simulink model "e9_sf_slswitch"  (R2020a)
settings: Solver=FixedStepAuto  StartTime=0.0  StopTime=options.T_train  FixedStep=options.dt  MaxStep=.2  RelTol=1e-3
model workspace (MAT data in the model file):
  PID_TRESH = 0.3
undefined symbols (not defined in the file or in its folder): DiscIntNeverNeededParam, options
libraries: neural x72, simulink x3
(part 3 of 3)

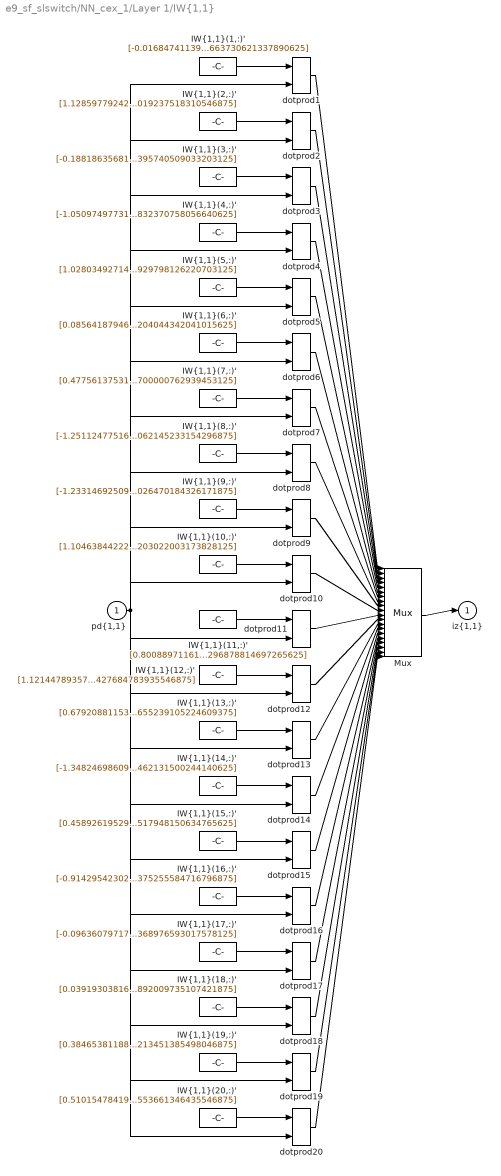
== system e9_sf_slswitch/NN_cex_1/Layer 1/IW{1,1} ==
  "pd{1,1}" : Inport  PortDimensions=6
      mask Display: e = 0.06;c1 = [120 230 180]/255;c2 = ([120 230 180]+0)/(256+128);c3 = ([120 230 180]+128)/(256+128);patch([0 1 1 0],[0 0 1 1],c1);patch([0 1 1 1-e 1-e 0+e],[0 0 1 1-e 0+e 0+e],c2);patch([0 0 1 1-e 0+e 0+e],[0 1 1 1-e 1-e 0+e],c3);plot([0 1 1 0 0],[0 0 1 1 0]);
  "IW{1,1}(1,:)'" : Constant  Value=[-0.0168474113906026019826800421697043930180370807647705078125;-1.0960190446116688800515248658484779298305511474609375;1.303822159020755488967324708937667310237884521484375;0.90483138367543614055676926000160165131092071533203125;-0.92904857435732768333735975829767994582653045654296875;0.7536625946512780505059936331235803663730621337890625]
      mask Display: e = 0.06;c1 = [120 150 230]/255;c2 = ([120 150 230]+0)/383;c3 = ([120 150 230]+128)/383;patch([0 1 1 0],[0 0 1 1],c1);patch([0 1 1 1-e 1-e 0+e],[0 0 1 1-e 0+e 0+e],c2);patch([0 0 1 1-e 0+e 0+e],[0 1 1 1-e 1-e 0+e],c3);plot([0 1 1 0 0],[0 0 1 1 0]);disp('Weights');
  "IW{1,1}(10,:)'" : Constant  Value=[1.104638442227569239406648193835280835628509521484375;-0.02443218271199705526885992412644554860889911651611328125;-0.54301394151020698775056416707229800522327423095703125;-2.64487319649380747677014369401149451732635498046875;0.83816378231433186218879427542560733854770660400390625;0.580117155258321748334537915070541203022003173828125]
      mask Display: e = 0.06;c1 = [120 150 230]/255;c2 = ([120 150 230]+0)/383;c3 = ([120 150 230]+128)/383;patch([0 1 1 0],[0 0 1 1],c1);patch([0 1 1 1-e 1-e 0+e],[0 0 1 1-e 0+e 0+e],c2);patch([0 0 1 1-e 0+e 0+e],[0 1 1 1-e 1-e 0+e],c3);plot([0 1 1 0 0],[0 0 1 1 0]);disp('Weights');
  "IW{1,1}(11,:)'" : Constant  Value=[0.80088971161301392154285849755979143083095550537109375;-1.4360458039470860303055133044836111366748809814453125;1.349244522904669896234963744063861668109893798828125;0.239507763293771269719201200132374651730060577392578125;-0.142625375011002863967490839058882556855678558349609375;-1.1145437179066368660329544582054950296878814697265625]
      mask Display: e = 0.06;c1 = [120 150 230]/255;c2 = ([120 150 230]+0)/383;c3 = ([120 150 230]+128)/383;patch([0 1 1 0],[0 0 1 1],c1);patch([0 1 1 1-e 1-e 0+e],[0 0 1 1-e 0+e 0+e],c2);patch([0 0 1 1-e 0+e 0+e],[0 1 1 1-e 1-e 0+e],c3);plot([0 1 1 0 0],[0 0 1 1 0]);disp('Weights');
  "IW{1,1}(12,:)'" : Constant  Value=[1.12144789357198959578454378060996532440185546875;-1.039431996259746693311853960040025413036346435546875;-0.06963854228211265040560107308920123614370822906494140625;-0.388663791726383378577480698368162848055362701416015625;-0.526178830323278834413258664426393806934356689453125;1.8227062352942435818903277322533540427684783935546875]
      mask Display: e = 0.06;c1 = [120 150 230]/255;c2 = ([120 150 230]+0)/383;c3 = ([120 150 230]+128)/383;patch([0 1 1 0],[0 0 1 1],c1);patch([0 1 1 1-e 1-e 0+e],[0 0 1 1-e 0+e 0+e],c2);patch([0 0 1 1-e 0+e 0+e],[0 1 1 1-e 1-e 0+e],c3);plot([0 1 1 0 0],[0 0 1 1 0]);disp('Weights');
  "IW{1,1}(13,:)'" : Constant  Value=[0.6792088115375027879139224751270376145839691162109375;-0.67422879238008082136701659692334942519664764404296875;1.1697043443831096620755261028534732758998870849609375;-0.5713364836554226666720524008269421756267547607421875;-1.3593652703803027481654908115160651504993438720703125;-0.67325667405921796326850881087011657655239105224609375]
      mask Display: e = 0.06;c1 = [120 150 230]/255;c2 = ([120 150 230]+0)/383;c3 = ([120 150 230]+128)/383;patch([0 1 1 0],[0 0 1 1],c1);patch([0 1 1 1-e 1-e 0+e],[0 0 1 1-e 0+e 0+e],c2);patch([0 0 1 1-e 0+e 0+e],[0 1 1 1-e 1-e 0+e],c3);plot([0 1 1 0 0],[0 0 1 1 0]);disp('Weights');
  "IW{1,1}(14,:)'" : Constant  Value=[-1.348246986096783839315094155608676373958587646484375;0.007208702054189595510858001858878196799196302890777587890625;0.689323370229841803080716999829746782779693603515625;0.274921664510416829951822137445560656487941741943359375;0.9517793019769207329972005027229897677898406982421875;1.4034991564643990447081023376085795462131500244140625]
      mask Display: e = 0.06;c1 = [120 150 230]/255;c2 = ([120 150 230]+0)/383;c3 = ([120 150 230]+128)/383;patch([0 1 1 0],[0 0 1 1],c1);patch([0 1 1 1-e 1-e 0+e],[0 0 1 1-e 0+e 0+e],c2);patch([0 0 1 1-e 0+e 0+e],[0 1 1 1-e 1-e 0+e],c3);plot([0 1 1 0 0],[0 0 1 1 0]);disp('Weights');
  "IW{1,1}(15,:)'" : Constant  Value=[0.458926195297770345149501736159436404705047607421875;-0.82721661614949237861793562842649407684803009033203125;-1.0472964443914991594652974526979960501194000244140625;2.286396458456293689920357792288996279239654541015625;-0.767283880026006226415802302653901278972625732421875;-1.2787583371301727286351024304167367517948150634765625]
      mask Display: e = 0.06;c1 = [120 150 230]/255;c2 = ([120 150 230]+0)/383;c3 = ([120 150 230]+128)/383;patch([0 1 1 0],[0 0 1 1],c1);patch([0 1 1 1-e 1-e 0+e],[0 0 1 1-e 0+e 0+e],c2);patch([0 0 1 1-e 0+e 0+e],[0 1 1 1-e 1-e 0+e],c3);plot([0 1 1 0 0],[0 0 1 1 0]);disp('Weights');
  "IW{1,1}(16,:)'" : Constant  Value=[-0.9142954230218294231491427126456983387470245361328125;1.086582668659030304070256534032523632049560546875;-0.5623194252036516349591011021402664482593536376953125;0.9130879165472227665389937101281248033046722412109375;-0.378624198635671704860072850351571105420589447021484375;1.1245605733918313529073884637909941375255584716796875]
      mask Display: e = 0.06;c1 = [120 150 230]/255;c2 = ([120 150 230]+0)/383;c3 = ([120 150 230]+128)/383;patch([0 1 1 0],[0 0 1 1],c1);patch([0 1 1 1-e 1-e 0+e],[0 0 1 1-e 0+e 0+e],c2);patch([0 0 1 1-e 0+e 0+e],[0 1 1 1-e 1-e 0+e],c3);plot([0 1 1 0 0],[0 0 1 1 0]);disp('Weights');
  "IW{1,1}(17,:)'" : Constant  Value=[-0.0963607971765284287979369537424645386636257171630859375;0.52383887892794100960003333966596983373165130615234375;1.1199200021715942643396601852145977318286895751953125;0.412214510505207132329275054871686734259128570556640625;1.493814360897363968661011313088238239288330078125;1.0969306752620930911490404469077475368976593017578125]
      mask Display: e = 0.06;c1 = [120 150 230]/255;c2 = ([120 150 230]+0)/383;c3 = ([120 150 230]+128)/383;patch([0 1 1 0],[0 0 1 1],c1);patch([0 1 1 1-e 1-e 0+e],[0 0 1 1-e 0+e 0+e],c2);patch([0 0 1 1-e 0+e 0+e],[0 1 1 1-e 1-e 0+e],c3);plot([0 1 1 0 0],[0 0 1 1 0]);disp('Weights');
  "IW{1,1}(18,:)'" : Constant  Value=[0.03919303816683929186925894327941932715475559234619140625;-1.705405108377961109766829395084641873836517333984375;1.4225063236010502265571631141938269138336181640625;0.74230993989574856062318986005266197025775909423828125;0.03172256129110760658473822104497230611741542816162109375;-0.64635944684935520143653775448910892009735107421875]
      mask Display: e = 0.06;c1 = [120 150 230]/255;c2 = ([120 150 230]+0)/383;c3 = ([120 150 230]+128)/383;patch([0 1 1 0],[0 0 1 1],c1);patch([0 1 1 1-e 1-e 0+e],[0 0 1 1-e 0+e 0+e],c2);patch([0 0 1 1-e 0+e 0+e],[0 1 1 1-e 1-e 0+e],c3);plot([0 1 1 0 0],[0 0 1 1 0]);disp('Weights');
  "IW{1,1}(19,:)'" : Constant  Value=[0.38465381188996261574430945984204299747943878173828125;-1.3456866197282078001506988584878854453563690185546875;1.0543182684732188558740517692058347165584564208984375;-1.09418022738094578016898594796657562255859375;0.381893554029432202856497724496875889599323272705078125;-0.96869250594760980543895811933907680213451385498046875]
      mask Display: e = 0.06;c1 = [120 150 230]/255;c2 = ([120 150 230]+0)/383;c3 = ([120 150 230]+128)/383;patch([0 1 1 0],[0 0 1 1],c1);patch([0 1 1 1-e 1-e 0+e],[0 0 1 1-e 0+e 0+e],c2);patch([0 0 1 1-e 0+e 0+e],[0 1 1 1-e 1-e 0+e],c3);plot([0 1 1 0 0],[0 0 1 1 0]);disp('Weights');
  "IW{1,1}(2,:)'" : Constant  Value=[1.1285977924294738894417378105572424829006195068359375;1.3719496232898198417871071796980686485767364501953125;-0.70013930920313305339419684969470836222171783447265625;-0.40779886428615153004528792735072784125804901123046875;-1.3652168438495941860111315691028721630573272705078125;-2.669548479833547371953272886457853019237518310546875]
      mask Display: e = 0.06;c1 = [120 150 230]/255;c2 = ([120 150 230]+0)/383;c3 = ([120 150 230]+128)/383;patch([0 1 1 0],[0 0 1 1],c1);patch([0 1 1 1-e 1-e 0+e],[0 0 1 1-e 0+e 0+e],c2);patch([0 0 1 1-e 0+e 0+e],[0 1 1 1-e 1-e 0+e],c3);plot([0 1 1 0 0],[0 0 1 1 0]);disp('Weights');
  "IW{1,1}(20,:)'" : Constant  Value=[0.51015478419691684397463404820882715284824371337890625;-0.797711507045957279871117862057872116565704345703125;-0.51591444607071179628832169328234158456325531005859375;-1.3440860874112698919446984291425906121730804443359375;1.16622740943395086787859327159821987152099609375;-1.0335932152524047733521683767321519553661346435546875]
      mask Display: e = 0.06;c1 = [120 150 230]/255;c2 = ([120 150 230]+0)/383;c3 = ([120 150 230]+128)/383;patch([0 1 1 0],[0 0 1 1],c1);patch([0 1 1 1-e 1-e 0+e],[0 0 1 1-e 0+e 0+e],c2);patch([0 0 1 1-e 0+e 0+e],[0 1 1 1-e 1-e 0+e],c3);plot([0 1 1 0 0],[0 0 1 1 0]);disp('Weights');
  "IW{1,1}(3,:)'" : Constant  Value=[-0.188186356814592503639005371951498091220855712890625;0.04608541339057010965962746240620617754757404327392578125;0.477858638180441774867546200766810216009616851806640625;-1.008508128728536679119542895932681858539581298828125;-1.2120727840960991983365602209232747554779052734375;-1.125534165151560461737290097516961395740509033203125]
      mask Display: e = 0.06;c1 = [120 150 230]/255;c2 = ([120 150 230]+0)/383;c3 = ([120 150 230]+128)/383;patch([0 1 1 0],[0 0 1 1],c1);patch([0 1 1 1-e 1-e 0+e],[0 0 1 1-e 0+e 0+e],c2);patch([0 0 1 1-e 0+e 0+e],[0 1 1 1-e 1-e 0+e],c3);plot([0 1 1 0 0],[0 0 1 1 0]);disp('Weights');
  "IW{1,1}(4,:)'" : Constant  Value=[-1.050974977312110869576144978054799139499664306640625;1.28629718055694386436016429797746241092681884765625;1.1326800600668465168752163663157261908054351806640625;-0.82019920554920144883936927726608701050281524658203125;0.13774083756492638830337682520621456205844879150390625;-0.7371803862906036730606729179271496832370758056640625]
      mask Display: e = 0.06;c1 = [120 150 230]/255;c2 = ([120 150 230]+0)/383;c3 = ([120 150 230]+128)/383;patch([0 1 1 0],[0 0 1 1],c1);patch([0 1 1 1-e 1-e 0+e],[0 0 1 1-e 0+e 0+e],c2);patch([0 0 1 1-e 0+e 0+e],[0 1 1 1-e 1-e 0+e],c3);plot([0 1 1 0 0],[0 0 1 1 0]);disp('Weights');
  "IW{1,1}(5,:)'" : Constant  Value=[1.0280349271452358106415658767218701541423797607421875;0.402195825930382111490501984008005820214748382568359375;-1.241108396864921470381659673876129090785980224609375;-1.0859758989406571583202776309917680919170379638671875;-0.98306862033537123490845033302321098744869232177734375;0.1483100282919010137749893374348175711929798126220703125]
      mask Display: e = 0.06;c1 = [120 150 230]/255;c2 = ([120 150 230]+0)/383;c3 = ([120 150 230]+128)/383;patch([0 1 1 0],[0 0 1 1],c1);patch([0 1 1 1-e 1-e 0+e],[0 0 1 1-e 0+e 0+e],c2);patch([0 0 1 1-e 0+e 0+e],[0 1 1 1-e 1-e 0+e],c3);plot([0 1 1 0 0],[0 0 1 1 0]);disp('Weights');
  "IW{1,1}(6,:)'" : Constant  Value=[0.08564187946235080062251654453575611114501953125;-1.0587143232822635585677062408649362623691558837890625;0.99533659624054260373071656431420706212520599365234375;1.348286797369088407805293172714300453662872314453125;-0.75350782154291906511645038335700519382953643798828125;-1.4647900005101688325481745778233744204044342041015625]
      mask Display: e = 0.06;c1 = [120 150 230]/255;c2 = ([120 150 230]+0)/383;c3 = ([120 150 230]+128)/383;patch([0 1 1 0],[0 0 1 1],c1);patch([0 1 1 1-e 1-e 0+e],[0 0 1 1-e 0+e 0+e],c2);patch([0 0 1 1-e 0+e 0+e],[0 1 1 1-e 1-e 0+e],c3);plot([0 1 1 0 0],[0 0 1 1 0]);disp('Weights');
  "IW{1,1}(7,:)'" : Constant  Value=[0.477561375317118452787923388314084149897098541259765625;-1.422656231024767681248022199724800884723663330078125;-0.34547470258236157025777401941013522446155548095703125;-0.6180573185750326548060229470138438045978546142578125;-1.103280002866290576690744273946620523929595947265625;-0.77979501040747056794799618728575296700000762939453125]
      mask Display: e = 0.06;c1 = [120 150 230]/255;c2 = ([120 150 230]+0)/383;c3 = ([120 150 230]+128)/383;patch([0 1 1 0],[0 0 1 1],c1);patch([0 1 1 1-e 1-e 0+e],[0 0 1 1-e 0+e 0+e],c2);patch([0 0 1 1-e 0+e 0+e],[0 1 1 1-e 1-e 0+e],c3);plot([0 1 1 0 0],[0 0 1 1 0]);disp('Weights');
  "IW{1,1}(8,:)'" : Constant  Value=[-1.251124775166029490236496712896041572093963623046875;1.0049111421650123165960621918202377855777740478515625;0.77937459336890635430705742692225612699985504150390625;-0.82407450496222856006767187864170409739017486572265625;0.380603729542155100329381411938811652362346649169921875;-1.18248664285082139002724943566136062145233154296875]
      mask Display: e = 0.06;c1 = [120 150 230]/255;c2 = ([120 150 230]+0)/383;c3 = ([120 150 230]+128)/383;patch([0 1 1 0],[0 0 1 1],c1);patch([0 1 1 1-e 1-e 0+e],[0 0 1 1-e 0+e 0+e],c2);patch([0 0 1 1-e 0+e 0+e],[0 1 1 1-e 1-e 0+e],c3);plot([0 1 1 0 0],[0 0 1 1 0]);disp('Weights');
  "IW{1,1}(9,:)'" : Constant  Value=[-1.2331469250970192863547936212853528559207916259765625;-0.2645454198128656120303503485047258436679840087890625;0.28872687215204162480830518688890151679515838623046875;-0.91218425882033937757142894042772240936756134033203125;-0.382274517593333584830617155603249557316303253173828125;1.50022977818130254235029497067444026470184326171875]
      mask Display: e = 0.06;c1 = [120 150 230]/255;c2 = ([120 150 230]+0)/383;c3 = ([120 150 230]+128)/383;patch([0 1 1 0],[0 0 1 1],c1);patch([0 1 1 1-e 1-e 0+e],[0 0 1 1-e 0+e 0+e],c2);patch([0 0 1 1-e 0+e 0+e],[0 1 1 1-e 1-e 0+e],c3);plot([0 1 1 0 0],[0 0 1 1 0]);disp('Weights');
  Mux : Mux  Inputs=20
      mask Display: e = 0.06;c1 = [120 150 230]/255;c2 = ([120 150 230]+0)/383;c3 = ([120 150 230]+128)/383;patch([0 1 1 0],[0 0 1 1],c1);patch([0 1 1 1-e 1-e 0+e],[0 0 1 1-e 0+e 0+e],c2);patch([0 0 1 1-e 0+e 0+e],[0 1 1 1-e 1-e 0+e],c3);plot([0 1 1 0 0],[0 0 1 1 0]);disp('Mux');
  dotprod{1..20} (20 alike) : neural/Weight Functions/dotprod
  "iz{1,1}" : Outport
      mask Display: e = 0.06;c1 = [120 230 180]/255;c2 = ([120 230 180]+0)/(256+128);c3 = ([120 230 180]+128)/(256+128);patch([0 1 1 0],[0 0 1 1],c1);patch([0 1 1 1-e 1-e 0+e],[0 0 1 1-e 0+e 0+e],c2);patch([0 0 1 1-e 0+e 0+e],[0 1 1 1-e 1-e 0+e],c3);plot([0 1 1 0 0],[0 0 1 1 0]);
  wires:
  "IW{1,1}(1,:)'"/1 -> dotprod1/1
  "pd{1,1}"/1 -> dotprod1/2, dotprod2/2, dotprod3/2, dotprod4/2, dotprod5/2, dotprod6/2, dotprod7/2, dotprod8/2, dotprod9/2, dotprod10/2, dotprod11/2, dotprod12/2, dotprod13/2, dotprod14/2, dotprod15/2, dotprod16/2, dotprod17/2, dotprod18/2, dotprod19/2, dotprod20/2
  dotprod1/1 -> Mux/1
  "IW{1,1}(2,:)'"/1 -> dotprod2/1
  dotprod2/1 -> Mux/2
  "IW{1,1}(3,:)'"/1 -> dotprod3/1
  dotprod3/1 -> Mux/3
  "IW{1,1}(4,:)'"/1 -> dotprod4/1
  dotprod4/1 -> Mux/4
  "IW{1,1}(5,:)'"/1 -> dotprod5/1
  dotprod5/1 -> Mux/5
  "IW{1,1}(6,:)'"/1 -> dotprod6/1
  dotprod6/1 -> Mux/6
  "IW{1,1}(7,:)'"/1 -> dotprod7/1
  dotprod7/1 -> Mux/7
  "IW{1,1}(8,:)'"/1 -> dotprod8/1
  dotprod8/1 -> Mux/8
  "IW{1,1}(9,:)'"/1 -> dotprod9/1
  dotprod9/1 -> Mux/9
  "IW{1,1}(10,:)'"/1 -> dotprod10/1
  dotprod10/1 -> Mux/10
  "IW{1,1}(11,:)'"/1 -> dotprod11/1
  dotprod11/1 -> Mux/11
  "IW{1,1}(12,:)'"/1 -> dotprod12/1
  dotprod12/1 -> Mux/12
  "IW{1,1}(13,:)'"/1 -> dotprod13/1
  dotprod13/1 -> Mux/13
  "IW{1,1}(14,:)'"/1 -> dotprod14/1
  dotprod14/1 -> Mux/14
  "IW{1,1}(15,:)'"/1 -> dotprod15/1
  dotprod15/1 -> Mux/15
  "IW{1,1}(16,:)'"/1 -> dotprod16/1
  dotprod16/1 -> Mux/16
  "IW{1,1}(17,:)'"/1 -> dotprod17/1
  dotprod17/1 -> Mux/17
  "IW{1,1}(18,:)'"/1 -> dotprod18/1
  dotprod18/1 -> Mux/18
  "IW{1,1}(19,:)'"/1 -> dotprod19/1
  dotprod19/1 -> Mux/19
  "IW{1,1}(20,:)'"/1 -> dotprod20/1
  dotprod20/1 -> Mux/20
  Mux/1 -> "iz{1,1}"/1

== system e9_sf_slswitch/NN_cex_1/Layer 2/Delays 1 ==
  "p{2}" : Inport  PortDimensions=20
      mask Display: e = 0.06;c1 = [120 230 180]/255;c2 = ([120 230 180]+0)/(256+128);c3 = ([120 230 180]+128)/(256+128);patch([0 1 1 0],[0 0 1 1],c1);patch([0 1 1 1-e 1-e 0+e],[0 0 1 1-e 0+e 0+e],c2);patch([0 0 1 1-e 0+e 0+e],[0 1 1 1-e 1-e 0+e],c3);plot([0 1 1 0 0],[0 0 1 1 0]);
  mux : Mux  Inputs=1
      mask Display: e = 0.06;c1 = [120 150 230]/255;c2 = ([120 150 230]+0)/383;c3 = ([120 150 230]+128)/383;patch([0 1 1 0],[0 0 1 1],c1);patch([0 1 1 1-e 1-e 0+e],[0 0 1 1-e 0+e 0+e],c2);patch([0 0 1 1-e 0+e 0+e],[0 1 1 1-e 1-e 0+e],c3);plot([0 1 1 0 0],[0 0 1 1 0]);disp('Mux')
  "pd{2,1}" : Outport
      mask Display: e = 0.06;c1 = [120 230 180]/255;c2 = ([120 230 180]+0)/(256+128);c3 = ([120 230 180]+128)/(256+128);patch([0 1 1 0],[0 0 1 1],c1);patch([0 1 1 1-e 1-e 0+e],[0 0 1 1-e 0+e 0+e],c2);patch([0 0 1 1-e 0+e 0+e],[0 1 1 1-e 1-e 0+e],c3);plot([0 1 1 0 0],[0 0 1 1 0]);
  wires:
  "p{2}"/1 -> mux/1
  mux/1 -> "pd{2,1}"/1

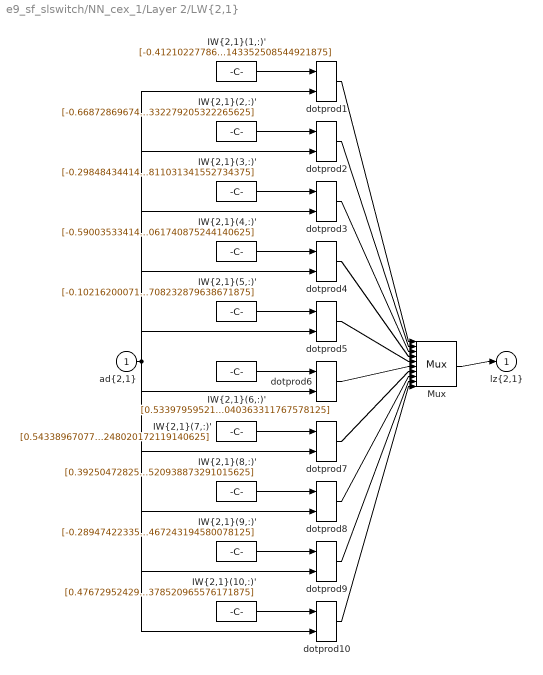
== system e9_sf_slswitch/NN_cex_1/Layer 2/LW{2,1} ==
  "ad{2,1}" : Inport  PortDimensions=20
      mask Display: e = 0.06;c1 = [120 230 180]/255;c2 = ([120 230 180]+0)/(256+128);c3 = ([120 230 180]+128)/(256+128);patch([0 1 1 0],[0 0 1 1],c1);patch([0 1 1 1-e 1-e 0+e],[0 0 1 1-e 0+e 0+e],c2);patch([0 0 1 1-e 0+e 0+e],[0 1 1 1-e 1-e 0+e],c3);plot([0 1 1 0 0],[0 0 1 1 0]);
  "IW{2,1}(1,:)'" : Constant  Value=[-0.412102277869951072464260732886032201349735260009765625;-0.0033102962537368790622849257232473973999731242656707763671875;0.498276475510173455507612061410327441990375518798828125;0.370594648987040031773432247064192779362201690673828125;-0.172702581187572423715437253122217953205108642578125;-0.28269873284898405785270369960926473140716552734375;0.1609017986261900567956928398416494019329547882080078125;0.57527437877796694376542063764645718038082122802734375;0.18571656848820394802856981186778284609317779541015625;-0.397447810976002013916286159656010568141937255859375;-0.49313231453008621318900850383215583860874176025390625;-0.3183651289608493417659929036744870245456695556640625;0.1503184907699568750860663612911594100296497344970703125;-0.343042617011638795165850979174138046801090240478515625;0.48159614366312475386422420342569239437580108642578125;-0.384340370033912359648553547231131233274936676025390625;0.319803972642864697828457565265125595033168792724609375;-0.169210525256166477436892137120594270527362823486328125;0.1082045460649214974058196503392537124454975128173828125;0.49225160804730883068458524576271884143352508544921875]
      mask Display: e = 0.06;c1 = [120 150 230]/255;c2 = ([120 150 230]+0)/383;c3 = ([120 150 230]+128)/383;patch([0 1 1 0],[0 0 1 1],c1);patch([0 1 1 1-e 1-e 0+e],[0 0 1 1-e 0+e 0+e],c2);patch([0 0 1 1-e 0+e 0+e],[0 1 1 1-e 1-e 0+e],c3);plot([0 1 1 0 0],[0 0 1 1 0]);disp('weights');
  "IW{2,1}(10,:)'" : Constant  Value=[0.476729524297248519193459515008726157248020172119140625;-0.407821347083386298582041717963875271379947662353515625;-0.2018949387792945693309576427054707892239093780517578125;-0.4059574043654183839180404902435839176177978515625;0.73472791573249873753326255609863437712192535400390625;0.511372507461387737492941596428863704204559326171875;0.69961983003993666319075828141649253666400909423828125;-0.234222692241623675624140332729439251124858856201171875;0.19033737019719054739397279263357631862163543701171875;-0.2296240379397176400999569523264653980731964111328125;0.52125524089998609422735853513586334884166717529296875;-0.95321599331459638815289281410514377057552337646484375;0.1506847813854093887098173354388563893735408782958984375;0.51547730872195796081314256298355758190155029296875;0.274123361606459725603457400211482308804988861083984375;0.1863257308692378988457249988641706295311450958251953125;-0.5345344958086812869879622667212970554828643798828125;0.2183490567687410288666427504722378216683864593505859375;-0.215592460422616927218086857465095818042755126953125;0.0175481619752120114597015998469942132942378520965576171875]
      mask Display: e = 0.06;c1 = [120 150 230]/255;c2 = ([120 150 230]+0)/383;c3 = ([120 150 230]+128)/383;patch([0 1 1 0],[0 0 1 1],c1);patch([0 1 1 1-e 1-e 0+e],[0 0 1 1-e 0+e 0+e],c2);patch([0 0 1 1-e 0+e 0+e],[0 1 1 1-e 1-e 0+e],c3);plot([0 1 1 0 0],[0 0 1 1 0]);disp('weights');
  "IW{2,1}(2,:)'" : Constant  Value=[-0.6687286967479215693543892484740354120731353759765625;0.53089310457156846378978798384196124970912933349609375;-0.00988650741851515406366512905833587865345180034637451171875;-0.16475866593556764971850725487456656992435455322265625;-0.83099792149795803641865177269210107624530792236328125;0.83286438268544260576931037576287053525447845458984375;-0.421930961865297604607150105948676355183124542236328125;0.06684041765297595028005872563880984671413898468017578125;-0.173504636537880951863144218805246055126190185546875;0.1793284238400363606036336250326712615787982940673828125;-0.412807134717095181031254469417035579681396484375;-0.1897621024386075549994501443507033400237560272216796875;0.1393131970130082886161204669406288303434848785400390625;0.1878438569324507312341410170120070688426494598388671875;0.86404371044378092125981538629275746643543243408203125;0.46470926606683515824869346033665351569652557373046875;0.038250058996138480704729545323061756789684295654296875;0.221752079748374464340798795092268846929073333740234375;0.192947140226262359163911241921596229076385498046875;-0.349200177440924852678705292419181205332279205322265625]
      mask Display: e = 0.06;c1 = [120 150 230]/255;c2 = ([120 150 230]+0)/383;c3 = ([120 150 230]+128)/383;patch([0 1 1 0],[0 0 1 1],c1);patch([0 1 1 1-e 1-e 0+e],[0 0 1 1-e 0+e 0+e],c2);patch([0 0 1 1-e 0+e 0+e],[0 1 1 1-e 1-e 0+e],c3);plot([0 1 1 0 0],[0 0 1 1 0]);disp('weights');
  "IW{2,1}(3,:)'" : Constant  Value=[-0.298484344147023239468552446851390413939952850341796875;0.190641928235647295508670140407048165798187255859375;0.1981536900428658432016248980289674364030361175537109375;-0.388862957242743612074065140404854901134967803955078125;0.21449537302792165416320813164929859340190887451171875;0.3863203233730050367711328362929634749889373779296875;0.68170524276259214513373763111303560435771942138671875;0.12950440289639064683768765462446026504039764404296875;0.327443722942501846961960154658299870789051055908203125;-0.542516816538905377598211998702026903629302978515625;0.3702632632852640437448599186609499156475067138671875;-0.262759426109619109723780638887546956539154052734375;0.398897950183966065740293061026022769510746002197265625;-0.2405628118556803751726391737975063733756542205810546875;-0.418319523738042098326417317366576753556728363037109375;-0.057500676569799409609817786304120090790092945098876953125;0.432838580152064944517320554950856603682041168212890625;0.406924514266054526689941894801449961960315704345703125;0.2437061579769842223353037979904911480844020843505859375;-0.451417764465296522669035539365722797811031341552734375]
      mask Display: e = 0.06;c1 = [120 150 230]/255;c2 = ([120 150 230]+0)/383;c3 = ([120 150 230]+128)/383;patch([0 1 1 0],[0 0 1 1],c1);patch([0 1 1 1-e 1-e 0+e],[0 0 1 1-e 0+e 0+e],c2);patch([0 0 1 1-e 0+e 0+e],[0 1 1 1-e 1-e 0+e],c3);plot([0 1 1 0 0],[0 0 1 1 0]);disp('weights');
  "IW{2,1}(4,:)'" : Constant  Value=[-0.590035334144344947304716697544790804386138916015625;-0.14251153895537560511996844070381484925746917724609375;0.055844163610838937206182208683458156883716583251953125;-0.25168425456298348930062047656974755227565765380859375;0.347940176225571440316031157635734416544437408447265625;0.334331889113240132704873985858284868299961090087890625;-0.3570468479858923682712656955118291079998016357421875;-0.487904252695575468834476851043291389942169189453125;0.066019736601342859927399331354536116123199462890625;0.09407698569578033798155303202292998321354389190673828125;-0.2450555949832949609312748862066655419766902923583984375;0.36422969241255109817956281403894536197185516357421875;-0.3245571948522207872400713313254527747631072998046875;0.64482395367362543847633560289978049695491790771484375;0.137767167812864410603168607849511317908763885498046875;0.429727741927319495385262371200951747596263885498046875;-0.043270745376913381796679658464199746958911418914794921875;0.14654430233835558095023543501156382262706756591796875;0.47476898943911083339486367549397982656955718994140625;0.55073672846336096942110316376783885061740875244140625]
      mask Display: e = 0.06;c1 = [120 150 230]/255;c2 = ([120 150 230]+0)/383;c3 = ([120 150 230]+128)/383;patch([0 1 1 0],[0 0 1 1],c1);patch([0 1 1 1-e 1-e 0+e],[0 0 1 1-e 0+e 0+e],c2);patch([0 0 1 1-e 0+e 0+e],[0 1 1 1-e 1-e 0+e],c3);plot([0 1 1 0 0],[0 0 1 1 0]);disp('weights');
  "IW{2,1}(5,:)'" : Constant  Value=[-0.1021620007108376970705876374267973005771636962890625;0.43940207024349131614826546865515410900115966796875;0.420315012299466383982604611446731723845005035400390625;-0.268809769837709711115536492798128165304660797119140625;-0.66491121568533506636100582909421063959598541259765625;0.81368602130842127007070985200698487460613250732421875;-0.0209290057054771945488358397824413259513676166534423828125;0.60030318645803582011666321704979054629802703857421875;0.05965638396169337109853358924738131463527679443359375;0.46479724467141825261506937749800272285938262939453125;-0.49210398709284419727083559337188489735126495361328125;-0.256405350236701135013817065555485896766185760498046875;0.2117572317136166837325816914017195813357830047607421875;0.0665783902974867725088614633932593278586864471435546875;-0.5574717002200204607476052842685021460056304931640625;-0.2042746665310815334937188936237362213432788848876953125;-0.3718070675272440173131371921044774353504180908203125;0.1607832109368834971885320328510715626180171966552734375;-0.09600919695738129033824037605882040224969387054443359375;-0.05362222814658224034900513288448564708232879638671875]
      mask Display: e = 0.06;c1 = [120 150 230]/255;c2 = ([120 150 230]+0)/383;c3 = ([120 150 230]+128)/383;patch([0 1 1 0],[0 0 1 1],c1);patch([0 1 1 1-e 1-e 0+e],[0 0 1 1-e 0+e 0+e],c2);patch([0 0 1 1-e 0+e 0+e],[0 1 1 1-e 1-e 0+e],c3);plot([0 1 1 0 0],[0 0 1 1 0]);disp('weights');
  "IW{2,1}(6,:)'" : Constant  Value=[0.533979595219758795821007879567332565784454345703125;0.4951544592086138951714247014024294912815093994140625;0.386181435740664991129733607522211968898773193359375;-0.421227567893845911140005000561359338462352752685546875;-0.25904069141159435929466781090013682842254638671875;0.05165911479104311199161969625492929480969905853271484375;-1.08656921433894648743034849758259952068328857421875;-0.38641003791316830273672167095355689525604248046875;-0.7472760361248951266333051535184495151042938232421875;-0.5552595613730793022710940931574441492557525634765625;-0.291988442597374942000243436268647201359272003173828125;0.207667673732985058610012174540315754711627960205078125;-0.0426652477493318915691133952350355684757232666015625;0.56286906728067720440122911895741708576679229736328125;0.1501150576296094996120444875487009994685649871826171875;0.17381267539819644785126229180605150759220123291015625;0.5555591475660615063958402970456518232822418212890625;0.423333454038131551389056994594284333288669586181640625;-0.118710432255852704752641102459165267646312713623046875;-0.11100521816291371302032331414011423476040363311767578125]
      mask Display: e = 0.06;c1 = [120 150 230]/255;c2 = ([120 150 230]+0)/383;c3 = ([120 150 230]+128)/383;patch([0 1 1 0],[0 0 1 1],c1);patch([0 1 1 1-e 1-e 0+e],[0 0 1 1-e 0+e 0+e],c2);patch([0 0 1 1-e 0+e 0+e],[0 1 1 1-e 1-e 0+e],c3);plot([0 1 1 0 0],[0 0 1 1 0]);disp('weights');
  "IW{2,1}(7,:)'" : Constant  Value=[0.54338967077317901210875561446300707757472991943359375;-0.84105172989018039952924254976096563041210174560546875;0.43087723858970339296803331308183260262012481689453125;-0.56782825305398720860949879352119751274585723876953125;0.58512476904167554092595082693151198327541351318359375;-0.55607002358524570961861854812013916671276092529296875;0.7576731872216970753441955821472220122814178466796875;0.029311043108750524377459356628605746664106845855712890625;0.92431422111959349319221246332745067775249481201171875;1.693240145772128446566284765140153467655181884765625;-0.94788635469439108671707572284503839910030364990234375;0.9062074408936997560459758460638113319873809814453125;0.1898811388872199412691799125241232104599475860595703125;0.412462918800584332768011108782957307994365692138671875;-1.7164187764461857899078722766716964542865753173828125;0.368384596456533153219226051078294403851032257080078125;-0.2457732347525502236695871260963031090795993804931640625;0.42101801253455750639886900899000465869903564453125;0.34679889467753233223135111984447576105594635009765625;0.362752559555652498435307506952085532248020172119140625]
      mask Display: e = 0.06;c1 = [120 150 230]/255;c2 = ([120 150 230]+0)/383;c3 = ([120 150 230]+128)/383;patch([0 1 1 0],[0 0 1 1],c1);patch([0 1 1 1-e 1-e 0+e],[0 0 1 1-e 0+e 0+e],c2);patch([0 0 1 1-e 0+e 0+e],[0 1 1 1-e 1-e 0+e],c3);plot([0 1 1 0 0],[0 0 1 1 0]);disp('weights');
  "IW{2,1}(8,:)'" : Constant  Value=[0.392504728252556056578015386548941023647785186767578125;-0.0225622009166554782222391395407612435519695281982421875;0.2449512161206320592921059642321779392659664154052734375;-0.054429114601580862176088970727505511604249477386474609375;0.66659271411129272788542721173143945634365081787109375;0.08788921988446192490318509271673974581062793731689453125;-0.3714667946322605107667413903982378542423248291015625;-0.1746532759190848882457913759935763664543628692626953125;-0.5943340620110413308196939397021196782588958740234375;-1.1628114657839889733992322362610138952732086181640625;0.34738617070303490219629338753293268382549285888671875;-0.57676721194810010029385693997028283774852752685546875;0.222745416942791429892878340979223139584064483642578125;0.254861092934894728490036186485667712986469268798828125;0.81439826381634594643088576049194671213626861572265625;0.7487022591524290504594318917952477931976318359375;0.30803198182668267701700415273080579936504364013671875;-0.079408889094169710087811608900665305554866790771484375;-0.44672250824831405413561924433452077209949493408203125;-0.60989804776822664766910975231439806520938873291015625]
      mask Display: e = 0.06;c1 = [120 150 230]/255;c2 = ([120 150 230]+0)/383;c3 = ([120 150 230]+128)/383;patch([0 1 1 0],[0 0 1 1],c1);patch([0 1 1 1-e 1-e 0+e],[0 0 1 1-e 0+e 0+e],c2);patch([0 0 1 1-e 0+e 0+e],[0 1 1 1-e 1-e 0+e],c3);plot([0 1 1 0 0],[0 0 1 1 0]);disp('weights');
  "IW{2,1}(9,:)'" : Constant  Value=[-0.28947422335969019702162086105090565979480743408203125;-0.40737358969895487437185011003748513758182525634765625;-0.225188131708673744402204874859307892620563507080078125;0.433840277621735215252130046792444773018360137939453125;-0.63533154521772072786944818290066905319690704345703125;0.1702495512060099025486437085419311188161373138427734375;0.042453738558729268992575356378438300453126430511474609375;-0.280841740829025965364706962645868770778179168701171875;0.312638313110935539551604733787826262414455413818359375;-0.479689671049607968544847835801192559301853179931640625;-0.496287994466178938868239356452249921858310699462890625;0.2659873939251600205579961766488850116729736328125;0.483536973285511206821496443808428011834621429443359375;-0.126263319200136392428390763598144985735416412353515625;-0.2367712373457120655917407248125527985394001007080078125;0.2870677995541661697842528155888430774211883544921875;0.2149413510902280222136795373444329015910625457763671875;0.34032619670570019021482721655047498643398284912109375;-0.222425782250009917984101548427133820950984954833984375;0.2176769002803791430711299881295417435467243194580078125]
      mask Display: e = 0.06;c1 = [120 150 230]/255;c2 = ([120 150 230]+0)/383;c3 = ([120 150 230]+128)/383;patch([0 1 1 0],[0 0 1 1],c1);patch([0 1 1 1-e 1-e 0+e],[0 0 1 1-e 0+e 0+e],c2);patch([0 0 1 1-e 0+e 0+e],[0 1 1 1-e 1-e 0+e],c3);plot([0 1 1 0 0],[0 0 1 1 0]);disp('weights');
  Mux : Mux  Inputs=10
      mask Display: e = 0.06;c1 = [120 150 230]/255;c2 = ([120 150 230]+0)/383;c3 = ([120 150 230]+128)/383;patch([0 1 1 0],[0 0 1 1],c1);patch([0 1 1 1-e 1-e 0+e],[0 0 1 1-e 0+e 0+e],c2);patch([0 0 1 1-e 0+e 0+e],[0 1 1 1-e 1-e 0+e],c3);plot([0 1 1 0 0],[0 0 1 1 0]);disp('Mux');
  dotprod{1..10} (10 alike) : neural/Weight Functions/dotprod
  "lz{2,1}" : Outport
      mask Display: e = 0.06;c1 = [120 230 180]/255;c2 = ([120 230 180]+0)/(256+128);c3 = ([120 230 180]+128)/(256+128);patch([0 1 1 0],[0 0 1 1],c1);patch([0 1 1 1-e 1-e 0+e],[0 0 1 1-e 0+e 0+e],c2);patch([0 0 1 1-e 0+e 0+e],[0 1 1 1-e 1-e 0+e],c3);plot([0 1 1 0 0],[0 0 1 1 0]);
  wires:
  "IW{2,1}(1,:)'"/1 -> dotprod1/1
  "ad{2,1}"/1 -> dotprod1/2, dotprod2/2, dotprod3/2, dotprod4/2, dotprod5/2, dotprod6/2, dotprod7/2, dotprod8/2, dotprod9/2, dotprod10/2
  dotprod1/1 -> Mux/1
  "IW{2,1}(2,:)'"/1 -> dotprod2/1
  dotprod2/1 -> Mux/2
  "IW{2,1}(3,:)'"/1 -> dotprod3/1
  dotprod3/1 -> Mux/3
  "IW{2,1}(4,:)'"/1 -> dotprod4/1
  dotprod4/1 -> Mux/4
  "IW{2,1}(5,:)'"/1 -> dotprod5/1
  dotprod5/1 -> Mux/5
  "IW{2,1}(6,:)'"/1 -> dotprod6/1
  dotprod6/1 -> Mux/6
  "IW{2,1}(7,:)'"/1 -> dotprod7/1
  dotprod7/1 -> Mux/7
  "IW{2,1}(8,:)'"/1 -> dotprod8/1
  dotprod8/1 -> Mux/8
  "IW{2,1}(9,:)'"/1 -> dotprod9/1
  dotprod9/1 -> Mux/9
  "IW{2,1}(10,:)'"/1 -> dotprod10/1
  dotprod10/1 -> Mux/10
  Mux/1 -> "lz{2,1}"/1

== system e9_sf_slswitch/NN_cex_1/Layer 3/Delays 1 ==
  "p{3}" : Inport  PortDimensions=10
      mask Display: e = 0.06;c1 = [120 230 180]/255;c2 = ([120 230 180]+0)/(256+128);c3 = ([120 230 180]+128)/(256+128);patch([0 1 1 0],[0 0 1 1],c1);patch([0 1 1 1-e 1-e 0+e],[0 0 1 1-e 0+e 0+e],c2);patch([0 0 1 1-e 0+e 0+e],[0 1 1 1-e 1-e 0+e],c3);plot([0 1 1 0 0],[0 0 1 1 0]);
  mux : Mux  Inputs=1
      mask Display: e = 0.06;c1 = [120 150 230]/255;c2 = ([120 150 230]+0)/383;c3 = ([120 150 230]+128)/383;patch([0 1 1 0],[0 0 1 1],c1);patch([0 1 1 1-e 1-e 0+e],[0 0 1 1-e 0+e 0+e],c2);patch([0 0 1 1-e 0+e 0+e],[0 1 1 1-e 1-e 0+e],c3);plot([0 1 1 0 0],[0 0 1 1 0]);disp('Mux')
  "pd{3,2}" : Outport
      mask Display: e = 0.06;c1 = [120 230 180]/255;c2 = ([120 230 180]+0)/(256+128);c3 = ([120 230 180]+128)/(256+128);patch([0 1 1 0],[0 0 1 1],c1);patch([0 1 1 1-e 1-e 0+e],[0 0 1 1-e 0+e 0+e],c2);patch([0 0 1 1-e 0+e 0+e],[0 1 1 1-e 1-e 0+e],c3);plot([0 1 1 0 0],[0 0 1 1 0]);
  wires:
  "p{3}"/1 -> mux/1
  mux/1 -> "pd{3,2}"/1

== system e9_sf_slswitch/NN_cex_1/Layer 3/LW{3,2} ==
  "ad{3,2}" : Inport  PortDimensions=10
      mask Display: e = 0.06;c1 = [120 230 180]/255;c2 = ([120 230 180]+0)/(256+128);c3 = ([120 230 180]+128)/(256+128);patch([0 1 1 0],[0 0 1 1],c1);patch([0 1 1 1-e 1-e 0+e],[0 0 1 1-e 0+e 0+e],c2);patch([0 0 1 1-e 0+e 0+e],[0 1 1 1-e 1-e 0+e],c3);plot([0 1 1 0 0],[0 0 1 1 0]);
  "IW{3,2}(1,:)'" : Constant  Value=[0.405983533651020189747526956125511787831783294677734375;-0.83585377193209586810240807608352042734622955322265625;-0.3998101917034249108695576069294475018978118896484375;-0.7497702463484821056027840313618071377277374267578125;-0.71460115427750359184955186719889752566814422607421875;0.48166786695840657639422488500713370740413665771484375;-1.817605188971331831027100633946247398853302001953125;0.68727286665727371772760534440749324858188629150390625;-1.1819455148445239256460581600549630820751190185546875;0.64901329601656165824152822096948511898517608642578125]
      mask Display: e = 0.06;c1 = [120 150 230]/255;c2 = ([120 150 230]+0)/383;c3 = ([120 150 230]+128)/383;patch([0 1 1 0],[0 0 1 1],c1);patch([0 1 1 1-e 1-e 0+e],[0 0 1 1-e 0+e 0+e],c2);patch([0 0 1 1-e 0+e 0+e],[0 1 1 1-e 1-e 0+e],c3);plot([0 1 1 0 0],[0 0 1 1 0]);disp('weights');
  Mux : Mux  Inputs=1
      mask Display: e = 0.06;c1 = [120 150 230]/255;c2 = ([120 150 230]+0)/383;c3 = ([120 150 230]+128)/383;patch([0 1 1 0],[0 0 1 1],c1);patch([0 1 1 1-e 1-e 0+e],[0 0 1 1-e 0+e 0+e],c2);patch([0 0 1 1-e 0+e 0+e],[0 1 1 1-e 1-e 0+e],c3);plot([0 1 1 0 0],[0 0 1 1 0]);disp('Mux');
  dotprod1 : neural/Weight Functions/dotprod
  "lz{3,2}" : Outport
      mask Display: e = 0.06;c1 = [120 230 180]/255;c2 = ([120 230 180]+0)/(256+128);c3 = ([120 230 180]+128)/(256+128);patch([0 1 1 0],[0 0 1 1],c1);patch([0 1 1 1-e 1-e 0+e],[0 0 1 1-e 0+e 0+e],c2);patch([0 0 1 1-e 0+e 0+e],[0 1 1 1-e 1-e 0+e],c3);plot([0 1 1 0 0],[0 0 1 1 0]);
  wires:
  "IW{3,2}(1,:)'"/1 -> dotprod1/1
  "ad{3,2}"/1 -> dotprod1/2
  dotprod1/1 -> Mux/1
  Mux/1 -> "lz{3,2}"/1

== stateflow chart e9_sf_slswitch/SwitchingController ==
  state STEADY
    entry: u = 0;
  state P
    du:
    u = p_control(e);
    state u = p_control(e) [function]
  state PID
    du:
    u = pid_control(e);
    state u = pid_control(e) [function]
  (default) -> STEADY
  STEADY -> P : [e > 0.01]
  P -> PID : [e < PID_TRESH]
  data: e function_input; u function_output; e function_input; u function_output; e input; u output double; PID output boolean; PID_TRESH parameter; P output boolean
